simulink model "Digital Protection - Instantaneous Overcurrent Element SLG Simulink"  (R2024b)
settings: Solver=ode4  StartTime=0.0  StopTime=1  FixedStep=1e-5  RelTol=1e-4
undefined symbols (not defined in the file): D1, Delta, dspblkCoreblockFVToolHelper, gcbh, rvar
libraries: spsThreePhaseBreakerLib x6, dspfdesign x6, powerlib_extras x6, simulink_extras x6, spsLoadFlowBusLib x4, spsThreePhaseVIMeasurementLib x4, spsDistributedParametersLineLib x3, spsThreePhaseSeriesRLCLoadLib x3, spsGroundLib x3, spsThreePhaseSeriesRLCBranchLib x2, spsSeriesRLCBranchLib x2, spsThreePhaseTransformerTwoWindingsLib x1
(part 2 of 2)

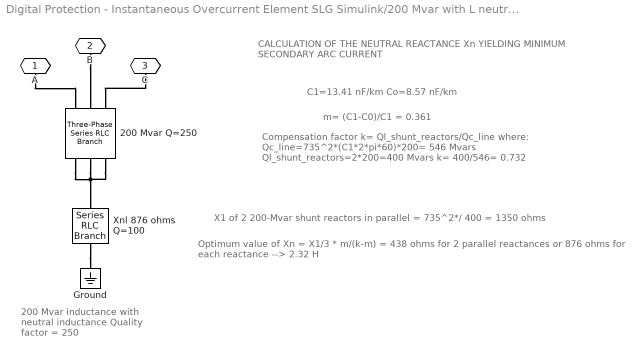
== system Digital Protection - Instantaneous Overcurrent Element SLG Simulink/200 Mvar with L neutral ==
  note: 200 Mvar inductance
      | with neutral inductance
      | Quality factor = 250
  note: C1=13.41 nF/km Co=8.57 nF/km
  note: m= (C1-C0)/C1 = 0.361
  note: Compensation factor k= Ql_shunt_reactors/Qc_line
      | where:
      |  Qc_line=735^2*(C1*2*pi*60)*200= 546 Mvars
      |  Ql_shunt_reactors=2*200=400 Mvars
      | k= 400/546= 0.732
  note: Optimum value of Xn = X1/3 * m/(k-m) = 438 ohms for 2 parallel reactances
      | or 876 ohms for each reactance --> 2.32 H
  note: X1 of 2 200-Mvar shunt reactors in parallel = 735^2*/ 400 = 1350 ohms
  note: CALCULATION OF THE NEUTRAL REACTANCE Xn
      | YIELDING MINIMUM SECONDARY ARC CURRENT
  200 Mvar Q=250 : spsThreePhaseSeriesRLCBranchLib/Three-Phase Series RLC Branch  LConnTagsString=A|B|C  RConnTagsString=A|B|C  BranchType=RL  Resistance=735^2/200/250  Inductance=735^2/200/377  Capacitance=1.0  Measurements=None
  Ground : spsGroundLib/Ground  LConnTagsString=a
  Xnl 876 ohms Q=100 : spsSeriesRLCBranchLib/Series RLC Branch  LConnTagsString=__new0  RConnTagsString=__new0  BranchType=RL  Resistance=876/100  Inductance=876/377  SetiL0=off  InitialCurrent=0  Capacitance=1.0  Setx0=off  InitialVoltage=0  Measurements=None
  A : PMIOPort  Side=Left
  B : PMIOPort  Port=2  Side=Left
  C : PMIOPort  Port=3  Side=Left
  connections:
  Xnl 876 ohms Q=100/RConn1 -- Ground/LConn1
  200 Mvar Q=250/RConn3 -- 200 Mvar Q=250/RConn2 -- Xnl 876 ohms Q=100/LConn1 -- 200 Mvar Q=250/RConn1
  C/RConn1 -- 200 Mvar Q=250/LConn3
  B/RConn1 -- 200 Mvar Q=250/LConn2
  A/RConn1 -- 200 Mvar Q=250/LConn1

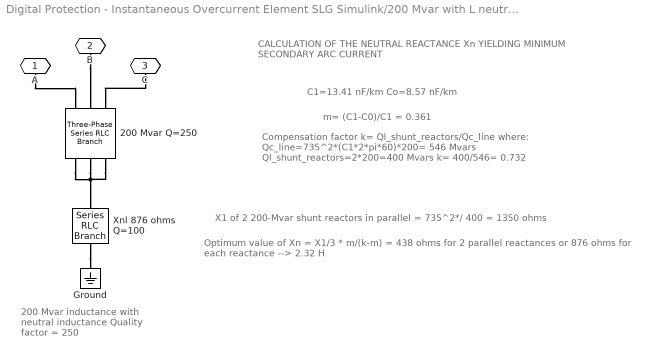
== system Digital Protection - Instantaneous Overcurrent Element SLG Simulink/200 Mvar with L neutral  ==
  note: CALCULATION OF THE NEUTRAL REACTANCE Xn
      | YIELDING MINIMUM SECONDARY ARC CURRENT
  note: X1 of 2 200-Mvar shunt reactors in parallel = 735^2*/ 400 = 1350 ohms
  note: Optimum value of Xn = X1/3 * m/(k-m) = 438 ohms for 2 parallel reactances
      | or 876 ohms for each reactance --> 2.32 H
  note: Compensation factor k= Ql_shunt_reactors/Qc_line
      | where:
      |  Qc_line=735^2*(C1*2*pi*60)*200= 546 Mvars
      |  Ql_shunt_reactors=2*200=400 Mvars
      | k= 400/546= 0.732
  note: m= (C1-C0)/C1 = 0.361
  note: C1=13.41 nF/km Co=8.57 nF/km
  note: 200 Mvar inductance
      | with neutral inductance
      | Quality factor = 250
  200 Mvar Q=250 : spsThreePhaseSeriesRLCBranchLib/Three-Phase Series RLC Branch  LConnTagsString=A|B|C  RConnTagsString=A|B|C  BranchType=RL  Resistance=735^2/200/250  Inductance=735^2/200/377  Capacitance=1.0  Measurements=None
  Ground : spsGroundLib/Ground  LConnTagsString=a
  Xnl 876 ohms Q=100 : spsSeriesRLCBranchLib/Series RLC Branch  LConnTagsString=__new0  RConnTagsString=__new0  BranchType=RL  Resistance=876/100  Inductance=876/377  SetiL0=off  InitialCurrent=0  Capacitance=1.0  Setx0=off  InitialVoltage=0  Measurements=None
  A : PMIOPort  Side=Left
  B : PMIOPort  Port=2  Side=Left
  C : PMIOPort  Port=3  Side=Left
  connections:
  A/RConn1 -- 200 Mvar Q=250/LConn1
  B/RConn1 -- 200 Mvar Q=250/LConn2
  C/RConn1 -- 200 Mvar Q=250/LConn3
  200 Mvar Q=250/RConn3 -- 200 Mvar Q=250/RConn2 -- Xnl 876 ohms Q=100/LConn1 -- 200 Mvar Q=250/RConn1
  Xnl 876 ohms Q=100/RConn1 -- Ground/LConn1

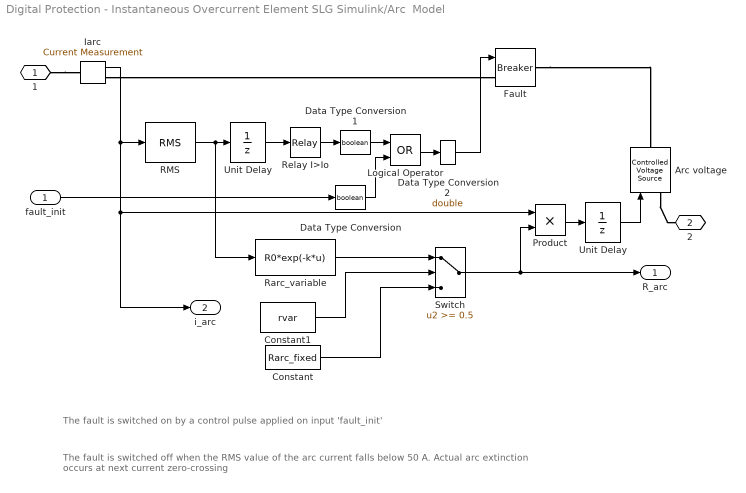
== system Digital Protection - Instantaneous Overcurrent Element SLG Simulink/Arc  Model ==
  note: The fault is switched on by a control pulse applied on input 'fault_init'
  note: The fault is switched off when the RMS value of the arc current falls below  50 A.
      | Actual arc extinction occurs at next current zero-crossing
  fault_init : Inport
  Arc voltage : spsControlledVoltageSourceLib/Controlled Voltage Source  Description=source block  Initialize=on  Source_Type=AC  Amplitude=0  Phase=0  Frequency=0  Measurements=None
      settings: AttributesFormatString=\n
  Constant : Constant  Value=Rarc_fixed
  Constant1 : Constant  Value=rvar
  Data Type Conversion : DataTypeConversion  OutDataTypeStr=boolean
  Data Type Conversion1 : DataTypeConversion  OutDataTypeStr=boolean
  Data Type Conversion2 : DataTypeConversion  OutDataTypeStr=double
  Fault : spsBreakerLib/Breaker  InitialState=0  SwitchingTimes="[ 4/60  5/60 ]"  External=on  BreakerResistance=.001  SnubberResistance=inf  SnubberCapacitance=0  Measurements=None  MoreParameters=off  NoBreakLoop=off
      settings: AttributesFormatString=\n
  Iarc : spsCurrentMeasurementLib/Current Measurement  Tag=PoWeRsYsTeMmEaSuReMeNt  PhasorSimulation=off  OutputType=Magnitude  PSBequivalent=0
      settings: AttributesFormatString=\n
  Logical Operator : Logic  Operator=OR
  Product : Product  InputSameDT=on  SaturateOnIntegerOverflow=on  OutDataTypeStr=Inherit: Same as first input
  RMS : spsRMSLib/RMS  TrueRMS=on  Freq=60  RMSInit=0  Ts=50e-6
  Rarc_variable : Fcn  Expr=R0*exp(-k*u)
  Relay I>Io : Relay  OnSwitchValue=I0*1.2  OffSwitchValue=I0  ZeroCross=off
  Switch : Switch  Threshold=0.5  ZeroCross=off  SaturateOnIntegerOverflow=off
  Unit Delay : UnitDelay  SampleTime=Ts  HasFrameUpgradeWarning=on
  "Unit Delay " : UnitDelay  SampleTime=Ts  HasFrameUpgradeWarning=on
  1 : PMIOPort  Side=Left
  2 : PMIOPort  Port=2  Side=Right
  R_arc : Outport  VectorParamsAs1DForOutWhenUnconnected=off
  i_arc : Outport  Port=2  VectorParamsAs1DForOutWhenUnconnected=off
  wires:
  RMS/1 -> "Unit Delay "/1, Rarc_variable/1
  Rarc_variable/1 -> Switch/1
  Switch/1 -> Product/2, R_arc/1
  Constant/1 -> Switch/3
  Constant1/1 -> Switch/2
  Product/1 -> Unit Delay/1
  "Unit Delay "/1 -> Relay I>Io/1
  fault_init/1 -> Data Type Conversion/1
  Data Type Conversion/1 -> Logical Operator/2
  Relay I>Io/1 -> Data Type Conversion1/1
  Data Type Conversion1/1 -> Logical Operator/1
  Logical Operator/1 -> Data Type Conversion2/1
  Iarc/1 -> RMS/1, Product/1, i_arc/1
  Unit Delay/1 -> Arc voltage/1
  Data Type Conversion2/1 -> Fault/1
  connections:
  1/RConn1 -- Iarc/LConn1
  Iarc/RConn1 -- Fault/LConn1
  Arc voltage/LConn1 -- 2/RConn1
  Fault/RConn1 -- Arc voltage/RConn1

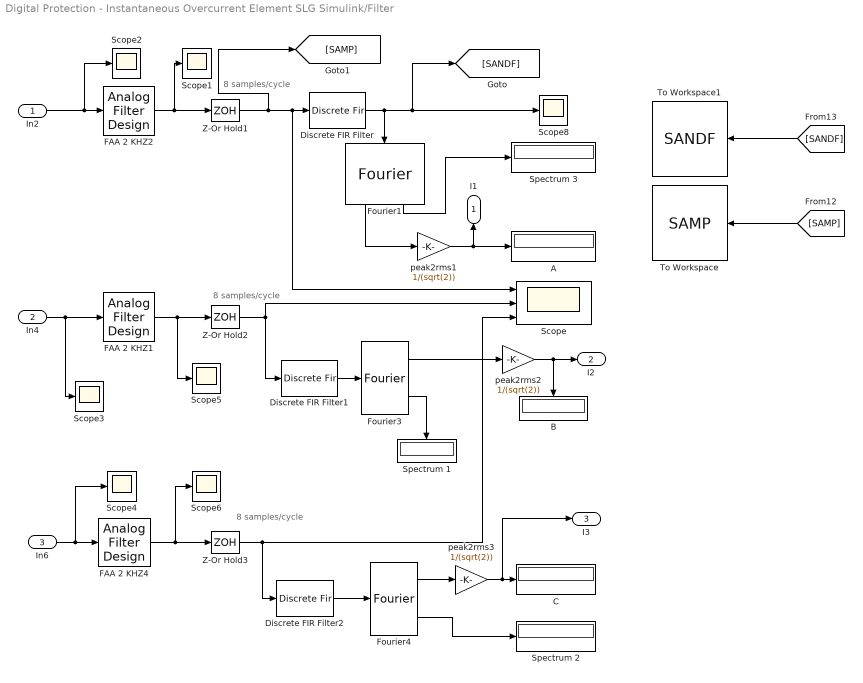
== system Digital Protection - Instantaneous Overcurrent Element SLG Simulink/Filter ==
  note: 8 samples/cycle
  note: 8 samples/cycle
  note: 8 samples/cycle
  In2 : Inport
  In4 : Inport  Port=2
  In6 : Inport  Port=3
  "A " : Display
  B : Display
  C : Display
  Discrete FIR Filter : DiscreteFir  LoadFcn=dspblkCoreblockFVToolHelper(gcbh,'load');  Coefficients=[-0.0186094 -0.0236782 -0.0307391 -0.0185278 0.0274259 0.1023722 0.1816244 0.2325969 0.2325969 0.1816244 0.1023722 0.0274259 -0.0185278 -0.0307391 -0.0236782 -0.0186094]
      settings: CopyFcn=dspblkCoreblockFVToolHelper(gcbh,'copy');  DeleteFcn=dspblkCoreblockFVToolHelper(gcbh,'close');  ModelCloseFcn=dspblkCoreblockFVToolHelper(gcbh,'close');  PreSaveFcn=dspblkCoreblockFVToolHelper(gcbh,'presave');  PostSaveFcn=dspblkCoreblockFVToolHelper(gcbh,'postsave');  CloseFcn=dspblkCoreblockFVToolHelper(gcbh,'close');
  Discrete FIR Filter1 : DiscreteFir  LoadFcn=dspblkCoreblockFVToolHelper(gcbh,'load');  Coefficients=[-0.0186094 -0.0236782 -0.0307391 -0.0185278 0.0274259 0.1023722 0.1816244 0.2325969 0.2325969 0.1816244 0.1023722 0.0274259 -0.0185278 -0.0307391 -0.0236782 -0.0186094]
      settings: CopyFcn=dspblkCoreblockFVToolHelper(gcbh,'copy');  DeleteFcn=dspblkCoreblockFVToolHelper(gcbh,'close');  ModelCloseFcn=dspblkCoreblockFVToolHelper(gcbh,'close');  PreSaveFcn=dspblkCoreblockFVToolHelper(gcbh,'presave');  PostSaveFcn=dspblkCoreblockFVToolHelper(gcbh,'postsave');  CloseFcn=dspblkCoreblockFVToolHelper(gcbh,'close');
  Discrete FIR Filter2 : DiscreteFir  LoadFcn=dspblkCoreblockFVToolHelper(gcbh,'load');  Coefficients=[-0.0186094 -0.0236782 -0.0307391 -0.0185278 0.0274259 0.1023722 0.1816244 0.2325969 0.2325969 0.1816244 0.1023722 0.0274259 -0.0185278 -0.0307391 -0.0236782 -0.0186094]
      settings: CopyFcn=dspblkCoreblockFVToolHelper(gcbh,'copy');  DeleteFcn=dspblkCoreblockFVToolHelper(gcbh,'close');  ModelCloseFcn=dspblkCoreblockFVToolHelper(gcbh,'close');  PreSaveFcn=dspblkCoreblockFVToolHelper(gcbh,'presave');  PostSaveFcn=dspblkCoreblockFVToolHelper(gcbh,'postsave');  CloseFcn=dspblkCoreblockFVToolHelper(gcbh,'close');
  FAA 2 KHZ1 : dspfdesign/Analog Filter Design  method=Butterworth  filttype=Lowpass  N=2  Wlo=2*pi*360  Whi=80  Rp=2  Rs=40
  FAA 2 KHZ2 : dspfdesign/Analog Filter Design  method=Butterworth  filttype=Lowpass  N=2  Wlo=2*pi*360  Whi=80  Rp=2  Rs=40
  FAA 2 KHZ4 : dspfdesign/Analog Filter Design  method=Butterworth  filttype=Lowpass  N=2  Wlo=2*pi*360  Whi=80  Rp=2  Rs=40
  Fourier1 : powerlib_extras/Measurements/Fourier  f1=60  n=1
  Fourier3 : powerlib_extras/Measurements/Fourier  f1=60  n=1
  Fourier4 : powerlib_extras/Measurements/Fourier  f1=60  n=1
  Scope : Scope  NumInputPorts=3
  Scope{1..6,8} (7 alike) : Scope
  Spectrum 1 : Display
  Spectrum 2 : Display
  Spectrum 3 : Display
  To Workspace : ToWorkspace  VariableName=SAMP  SaveFormat=Timeseries  SampleTime=-1
  To Workspace1 : ToWorkspace  VariableName=SANDF  SaveFormat=Timeseries  SampleTime=-1
  Z-Or Hold1 : ZeroOrderHold  SampleTime=0.002
  Z-Or Hold2 : ZeroOrderHold  SampleTime=0.002
  Z-Or Hold3 : ZeroOrderHold  SampleTime=0.002
  peak2rms1 : Gain  Gain=1/(sqrt(2))  SaturateOnIntegerOverflow=on  OutDataTypeStr=Inherit: Same as input  ParamDataTypeStr=Inherit: Same as input
  peak2rms2 : Gain  Gain=1/(sqrt(2))  SaturateOnIntegerOverflow=on  OutDataTypeStr=Inherit: Same as input  ParamDataTypeStr=Inherit: Same as input
  peak2rms3 : Gain  Gain=1/(sqrt(2))  SaturateOnIntegerOverflow=on  OutDataTypeStr=Inherit: Same as input  ParamDataTypeStr=Inherit: Same as input
  I1 : Outport
  I2 : Outport  Port=2
  I3 : Outport  Port=3
  wires:
  In2/1 -> Scope2/1, FAA 2 KHZ2/1
  FAA 2 KHZ2/1 -> Scope1/1, Z-Or Hold1/1
  Fourier4/2 -> Spectrum 2/1
  Fourier3/2 -> Spectrum 1/1
  FAA 2 KHZ1/1 -> Z-Or Hold2/1, Scope5/1
  In4/1 -> Scope3/1, FAA 2 KHZ1/1
  FAA 2 KHZ4/1 -> Z-Or Hold3/1, Scope6/1
  In6/1 -> Scope4/1, FAA 2 KHZ4/1
  Fourier1/2 -> Spectrum 3/1
  Z-Or Hold1/1 -> [SAMP], Scope/1, Discrete FIR Filter/1
  Discrete FIR Filter/1 -> [SANDF], Scope8/1, Fourier1/1
  Discrete FIR Filter1/1 -> Fourier3/1
  Z-Or Hold3/1 -> Scope/3, Discrete FIR Filter2/1
  Discrete FIR Filter2/1 -> Fourier4/1
  Z-Or Hold2/1 -> Discrete FIR Filter1/1, Scope/2
  Fourier1/1 -> peak2rms1/1
  Fourier3/1 -> peak2rms2/1
  peak2rms3/1 -> I3/1, C/1
  peak2rms1/1 -> I1/1, "A "/1
  peak2rms2/1 -> I2/1, B/1
  Fourier4/1 -> peak2rms3/1
  [SANDF] -> To Workspace1/1
  [SAMP] -> To Workspace/1

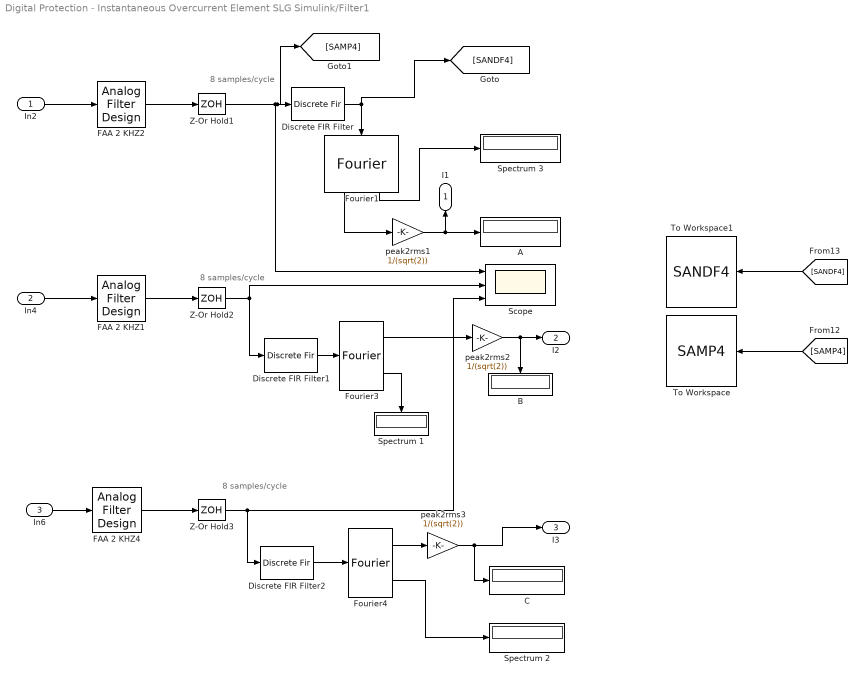
== system Digital Protection - Instantaneous Overcurrent Element SLG Simulink/Filter1 ==
  note: 8 samples/cycle
  note: 8 samples/cycle
  note: 8 samples/cycle
  In2 : Inport
  In4 : Inport  Port=2
  In6 : Inport  Port=3
  "A " : Display
  B : Display
  C : Display
  Discrete FIR Filter : DiscreteFir  LoadFcn=dspblkCoreblockFVToolHelper(gcbh,'load');  Coefficients=[-0.0186094 -0.0236782 -0.0307391 -0.0185278 0.0274259 0.1023722 0.1816244 0.2325969 0.2325969 0.1816244 0.1023722 0.0274259 -0.0185278 -0.0307391 -0.0236782 -0.0186094]
      settings: CopyFcn=dspblkCoreblockFVToolHelper(gcbh,'copy');  DeleteFcn=dspblkCoreblockFVToolHelper(gcbh,'close');  ModelCloseFcn=dspblkCoreblockFVToolHelper(gcbh,'close');  PreSaveFcn=dspblkCoreblockFVToolHelper(gcbh,'presave');  PostSaveFcn=dspblkCoreblockFVToolHelper(gcbh,'postsave');  CloseFcn=dspblkCoreblockFVToolHelper(gcbh,'close');
  Discrete FIR Filter1 : DiscreteFir  LoadFcn=dspblkCoreblockFVToolHelper(gcbh,'load');  Coefficients=[-0.0186094 -0.0236782 -0.0307391 -0.0185278 0.0274259 0.1023722 0.1816244 0.2325969 0.2325969 0.1816244 0.1023722 0.0274259 -0.0185278 -0.0307391 -0.0236782 -0.0186094]
      settings: CopyFcn=dspblkCoreblockFVToolHelper(gcbh,'copy');  DeleteFcn=dspblkCoreblockFVToolHelper(gcbh,'close');  ModelCloseFcn=dspblkCoreblockFVToolHelper(gcbh,'close');  PreSaveFcn=dspblkCoreblockFVToolHelper(gcbh,'presave');  PostSaveFcn=dspblkCoreblockFVToolHelper(gcbh,'postsave');  CloseFcn=dspblkCoreblockFVToolHelper(gcbh,'close');
  Discrete FIR Filter2 : DiscreteFir  LoadFcn=dspblkCoreblockFVToolHelper(gcbh,'load');  Coefficients=[-0.0186094 -0.0236782 -0.0307391 -0.0185278 0.0274259 0.1023722 0.1816244 0.2325969 0.2325969 0.1816244 0.1023722 0.0274259 -0.0185278 -0.0307391 -0.0236782 -0.0186094]
      settings: CopyFcn=dspblkCoreblockFVToolHelper(gcbh,'copy');  DeleteFcn=dspblkCoreblockFVToolHelper(gcbh,'close');  ModelCloseFcn=dspblkCoreblockFVToolHelper(gcbh,'close');  PreSaveFcn=dspblkCoreblockFVToolHelper(gcbh,'presave');  PostSaveFcn=dspblkCoreblockFVToolHelper(gcbh,'postsave');  CloseFcn=dspblkCoreblockFVToolHelper(gcbh,'close');
  FAA 2 KHZ1 : dspfdesign/Analog Filter Design  method=Butterworth  filttype=Lowpass  N=2  Wlo=2*pi*360  Whi=80  Rp=2  Rs=40
  FAA 2 KHZ2 : dspfdesign/Analog Filter Design  method=Butterworth  filttype=Lowpass  N=2  Wlo=2*pi*360  Whi=80  Rp=2  Rs=40
  FAA 2 KHZ4 : dspfdesign/Analog Filter Design  method=Butterworth  filttype=Lowpass  N=2  Wlo=2*pi*360  Whi=80  Rp=2  Rs=40
  Fourier1 : powerlib_extras/Measurements/Fourier  f1=60  n=1
  Fourier3 : powerlib_extras/Measurements/Fourier  f1=60  n=1
  Fourier4 : powerlib_extras/Measurements/Fourier  f1=60  n=1
  Scope : Scope  NumInputPorts=3
  Spectrum 1 : Display
  Spectrum 2 : Display
  Spectrum 3 : Display
  To Workspace : ToWorkspace  VariableName=SAMP4  SaveFormat=Timeseries  SampleTime=-1
  To Workspace1 : ToWorkspace  VariableName=SANDF4  SaveFormat=Timeseries  SampleTime=-1
  Z-Or Hold1 : ZeroOrderHold  SampleTime=0.002
  Z-Or Hold2 : ZeroOrderHold  SampleTime=0.002
  Z-Or Hold3 : ZeroOrderHold  SampleTime=0.002
  peak2rms1 : Gain  Gain=1/(sqrt(2))  SaturateOnIntegerOverflow=on  OutDataTypeStr=Inherit: Same as input  ParamDataTypeStr=Inherit: Same as input
  peak2rms2 : Gain  Gain=1/(sqrt(2))  SaturateOnIntegerOverflow=on  OutDataTypeStr=Inherit: Same as input  ParamDataTypeStr=Inherit: Same as input
  peak2rms3 : Gain  Gain=1/(sqrt(2))  SaturateOnIntegerOverflow=on  OutDataTypeStr=Inherit: Same as input  ParamDataTypeStr=Inherit: Same as input
  I1 : Outport
  I2 : Outport  Port=2
  I3 : Outport  Port=3
  wires:
  In2/1 -> FAA 2 KHZ2/1
  FAA 2 KHZ2/1 -> Z-Or Hold1/1
  Fourier4/2 -> Spectrum 2/1
  Fourier3/2 -> Spectrum 1/1
  FAA 2 KHZ1/1 -> Z-Or Hold2/1
  In4/1 -> FAA 2 KHZ1/1
  FAA 2 KHZ4/1 -> Z-Or Hold3/1
  In6/1 -> FAA 2 KHZ4/1
  Fourier1/2 -> Spectrum 3/1
  Z-Or Hold1/1 -> [SAMP4], Discrete FIR Filter/1, Scope/1
  Discrete FIR Filter1/1 -> Fourier3/1
  Z-Or Hold3/1 -> Scope/3, Discrete FIR Filter2/1
  Discrete FIR Filter2/1 -> Fourier4/1
  Z-Or Hold2/1 -> Discrete FIR Filter1/1, Scope/2
  Fourier1/1 -> peak2rms1/1
  Fourier3/1 -> peak2rms2/1
  peak2rms3/1 -> C/1, I3/1
  peak2rms1/1 -> I1/1, "A "/1
  peak2rms2/1 -> I2/1, B/1
  Fourier4/1 -> peak2rms3/1
  [SAMP4] -> To Workspace/1
  [SANDF4] -> To Workspace1/1
  Discrete FIR Filter/1 -> [SANDF4], Fourier1/1

== system Digital Protection - Instantaneous Overcurrent Element SLG Simulink/More Info ==

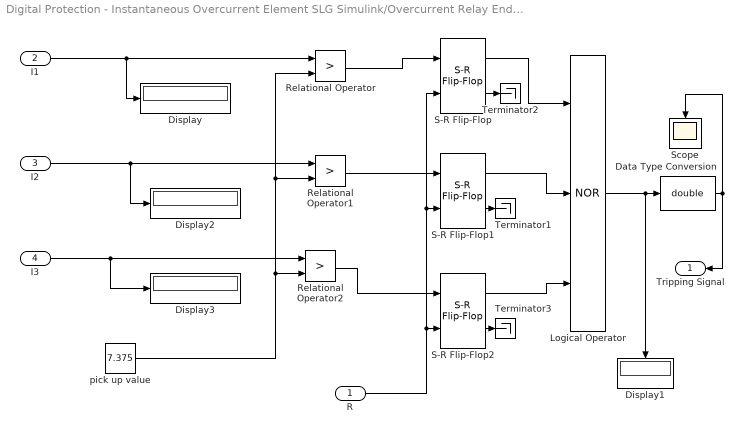
== system Digital Protection - Instantaneous Overcurrent Element SLG Simulink/Overcurrent Relay End 1  ==
  R : Inport
  I1 : Inport  Port=2
  I2 : Inport  Port=3
  I3 : Inport  Port=4
  Data Type Conversion : DataTypeConversion  OutDataTypeStr=double  SaturateOnIntegerOverflow=off  RndMeth=Floor
  Display{,1..3} (4 alike) : Display
  Logical Operator : Logic  Operator=NOR  Inputs=3  AllPortsSameDT=off  OutDataTypeStr=boolean
  Relational Operator : RelationalOperator  Operator=>  OutDataTypeStr=boolean  InputSameDT=off
  Relational Operator1 : RelationalOperator  Operator=>  OutDataTypeStr=boolean  InputSameDT=off
  Relational Operator2 : RelationalOperator  Operator=>  OutDataTypeStr=boolean  InputSameDT=off
  S-R Flip-Flop : simulink_extras/Flip Flops/S-R Flip-Flop  initial_condition=0
  S-R Flip-Flop1 : simulink_extras/Flip Flops/S-R Flip-Flop  initial_condition=0
  S-R Flip-Flop2 : simulink_extras/Flip Flops/S-R Flip-Flop  initial_condition=0
  Scope : Scope
  Terminator1 : Terminator
  Terminator2 : Terminator
  Terminator3 : Terminator
  pick up value : Constant  Value=7.375
  Tripping Signal : Outport  VectorParamsAs1DForOutWhenUnconnected=off
  wires:
  I1/1 -> Display/1, Relational Operator/1
  I2/1 -> Display2/1, Relational Operator1/1
  pick up value/1 -> Relational Operator/2, Relational Operator1/2, Relational Operator2/2
  Relational Operator/1 -> S-R Flip-Flop/1
  Relational Operator1/1 -> S-R Flip-Flop1/1
  Relational Operator2/1 -> S-R Flip-Flop2/1
  S-R Flip-Flop2/1 -> Logical Operator/3
  S-R Flip-Flop1/1 -> Logical Operator/2
  S-R Flip-Flop/1 -> Logical Operator/1
  Logical Operator/1 -> Display1/1, Data Type Conversion/1
  Data Type Conversion/1 -> Scope/1, Tripping Signal/1
  I3/1 -> Display3/1, Relational Operator2/1
  R/1 -> S-R Flip-Flop/2, S-R Flip-Flop1/2, S-R Flip-Flop2/2
  S-R Flip-Flop/2 -> Terminator2/1
  S-R Flip-Flop1/2 -> Terminator1/1
  S-R Flip-Flop2/2 -> Terminator3/1

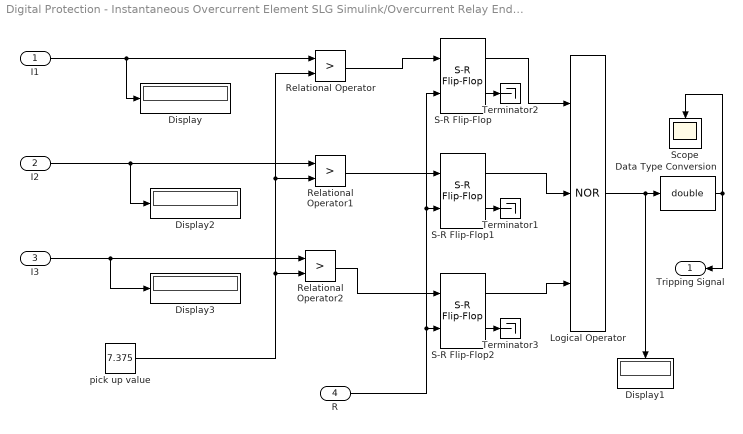
== system Digital Protection - Instantaneous Overcurrent Element SLG Simulink/Overcurrent Relay End 2 ==
  I1 : Inport
  I2 : Inport  Port=2
  I3 : Inport  Port=3
  R : Inport  Port=4
  Data Type Conversion : DataTypeConversion  OutDataTypeStr=double  SaturateOnIntegerOverflow=off  RndMeth=Floor
  Display{,1..3} (4 alike) : Display
  Logical Operator : Logic  Operator=NOR  Inputs=3  AllPortsSameDT=off  OutDataTypeStr=boolean
  Relational Operator : RelationalOperator  Operator=>  OutDataTypeStr=boolean  InputSameDT=off
  Relational Operator1 : RelationalOperator  Operator=>  OutDataTypeStr=boolean  InputSameDT=off
  Relational Operator2 : RelationalOperator  Operator=>  OutDataTypeStr=boolean  InputSameDT=off
  S-R Flip-Flop : simulink_extras/Flip Flops/S-R Flip-Flop  initial_condition=0
  S-R Flip-Flop1 : simulink_extras/Flip Flops/S-R Flip-Flop  initial_condition=0
  S-R Flip-Flop2 : simulink_extras/Flip Flops/S-R Flip-Flop  initial_condition=0
  Scope : Scope
  Terminator1 : Terminator
  Terminator2 : Terminator
  Terminator3 : Terminator
  pick up value : Constant  Value=7.375
  Tripping Signal : Outport  VectorParamsAs1DForOutWhenUnconnected=off
  wires:
  I1/1 -> Display/1, Relational Operator/1
  I2/1 -> Display2/1, Relational Operator1/1
  pick up value/1 -> Relational Operator/2, Relational Operator1/2, Relational Operator2/2
  Relational Operator/1 -> S-R Flip-Flop/1
  Relational Operator1/1 -> S-R Flip-Flop1/1
  Relational Operator2/1 -> S-R Flip-Flop2/1
  S-R Flip-Flop2/1 -> Logical Operator/3
  S-R Flip-Flop1/1 -> Logical Operator/2
  S-R Flip-Flop/1 -> Logical Operator/1
  Logical Operator/1 -> Display1/1, Data Type Conversion/1
  Data Type Conversion/1 -> Scope/1, Tripping Signal/1
  I3/1 -> Display3/1, Relational Operator2/1
  R/1 -> S-R Flip-Flop/2, S-R Flip-Flop1/2, S-R Flip-Flop2/2
  S-R Flip-Flop/2 -> Terminator2/1
  S-R Flip-Flop1/2 -> Terminator1/1
  S-R Flip-Flop2/2 -> Terminator3/1
